simulink model "c_ep_approx_bias"  (R2024b)
settings: Solver=VariableStepAuto  StartTime=0.0  StopTime=2000  RelTol=1e-3
settings Model: Creator=merlin  LastModifiedBy=merlin

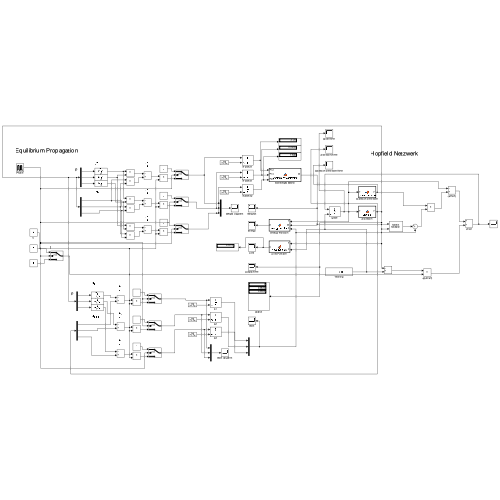
[thumbnail: Simulink's stored preview of the top-level diagram]
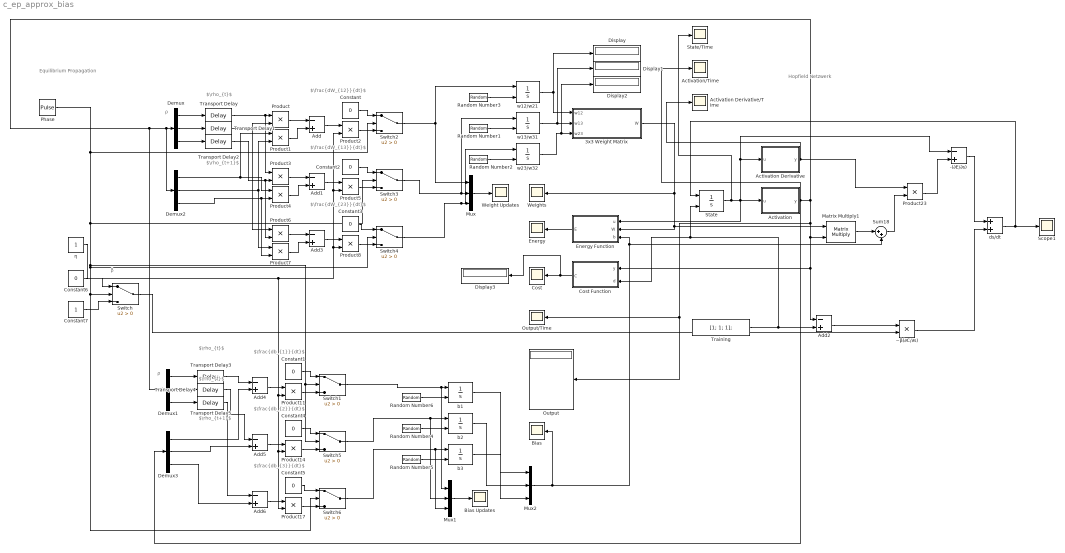
== system c_ep_approx_bias ==
  note: ρ
  note: β
  note: Equilibrium Propagation
  note: Hopfield Netzwerk
  note: $\frac{dW_{12}}{dt}$
  note: $\rho_{t}$
  note: $\rho_{t+1}$
  note: $\frac{dW_{13}}{dt}$
  note: $\frac{dW_{23}}{dt}$
  note: $\rho_{t}$
  note: $\frac{db_{2}}{dt}$
  note: ρ
  note: $\rho_{t+1}$
  note: $\frac{db_{1}}{dt}$
  note: $\frac{db_{3}}{dt}$
  note: $\rho_{t}$
  -(∂E/∂s) : Sum  Inputs=-+
  3x3 Weight Matrix : MATLAB Function  TreatAsAtomicUnit=on
  Activation : MATLAB Function  TreatAsAtomicUnit=on
  Activation Derivative : MATLAB Function  TreatAsAtomicUnit=on
  Activation Derivative/Time : Scope
  Activation/Time : Scope
  Add{,1..6} (7 alike) : Sum  Inputs=-+
  Bias : Scope
  Bias Updates : Scope
  Constant{,1..6} (7 alike) : Constant  Value=0
  Constant7 : Constant
  Cost : Scope
  Cost Function : MATLAB Function  TreatAsAtomicUnit=on
  Demux{,1..3} (4 alike) : Demux  Outputs=3
  Display{,1..3} (4 alike) : Display
  Energy : Scope
  Energy Function : MATLAB Function  TreatAsAtomicUnit=on
  Matrix Multiply1 : Product  Multiplication=Matrix(*)
  Mux : Mux  Inputs=3
  Mux1 : Mux  Inputs=3
  Mux2 : Mux  Inputs=3
  Output : Display
  Output/Time : Scope
  Phase : DiscretePulseGenerator  PulseType=Time based  Period=20  PulseWidth=50
  Product{,1..8,11,14,17,23} (13 alike) : Product
  Random Number1 : RandomNumber  Seed=13  SampleTime=0.1
  Random Number2 : RandomNumber  Seed=23  SampleTime=0.1
  Random Number3 : RandomNumber  Seed=12  SampleTime=0.1
  Random Number4 : RandomNumber  Seed=992  SampleTime=0.1
  Random Number5 : RandomNumber  Seed=993  SampleTime=0.1
  Random Number6 : RandomNumber  Seed=991  SampleTime=0.1
  Scope1 : Scope
  State : Integrator  InitialConditionSource=external
  State/Time : Scope
  Sum18 : Sum  Inputs=|++
  Switch{,1..6} (7 alike) : Switch  Criteria=u2 > Threshold  SaturateOnIntegerOverflow=off  InputSameDT=off
  Training : Constant  Value=[1; 1; 1];  VectorParams1D=off
  Transport Delay{,1..5} (6 alike) : TransportDelay
  Weight Updates : Scope
  Weights : Scope
  b1 : Integrator  InitialConditionSource=external
  b2 : Integrator  InitialConditionSource=external
  b3 : Integrator  InitialConditionSource=external
  ds/dt : Sum
  w12/w21 : Integrator  InitialConditionSource=external
  w13/w31 : Integrator  InitialConditionSource=external
  w23/w32 : Integrator  InitialConditionSource=external
  η : Constant
  −β(∂C/∂s) : Product
  wires:
  Constant6/1 -> Switch/1
  Constant7/1 -> Switch/3
  Phase/1 -> Switch6/2, Switch/2, Switch4/2, Switch5/2, Switch1/2, Switch3/2, Switch2/2
  Product23/1 -> -(∂E/∂s)/2
  Energy Function/1(E) -> Energy/1
  −β(∂C/∂s)/1 -> ds/dt/2
  Cost Function/1(C) -> Display3/1, Cost/1
  3x3 Weight Matrix/1(W) -> Weights/1, Energy Function/2(W), Matrix Multiply1/1
  w12/w21/1 -> 3x3 Weight Matrix/1(w12), Display/1
  ds/dt/1 -> Scope1/1, State/1
  Training/1 -> Cost Function/2(d), State/2, Add2/2
  -(∂E/∂s)/1 -> ds/dt/1
  Add2/1 -> −β(∂C/∂s)/1
  Sum18/1 -> Product23/2
  Matrix Multiply1/1 -> Sum18/1
  Activation Derivative/1(y) -> Activation Derivative/Time/1, Product23/1
  State/1 -> State/Time/1, Activation/1(u), Energy Function/1(u), -(∂E/∂s)/1, Activation Derivative/1(u)
  Activation/1(y) -> Demux3/1, Add2/1, Cost Function/1(y), Matrix Multiply1/2, Output/1, Output/Time/1, Demux2/1, Demux/1, Demux1/1, Activation/Time/1
  Switch/1 -> −β(∂C/∂s)/2
  w13/w31/1 -> Display1/1, 3x3 Weight Matrix/2(w13)
  w23/w32/1 -> Display2/1, 3x3 Weight Matrix/3(w23)
  Mux/1 -> Weight Updates/1
  Demux/1 -> Transport Delay/1
  Demux/2 -> Transport Delay1/1
  Demux/3 -> Transport Delay2/1
  η/1 -> Product5/2, Product2/2, Product8/2, Product17/2, Product14/2, Product11/2
  Product/1 -> Add/1
  Product1/1 -> Add/2
  Add/1 -> Product2/1
  Product2/1 -> Switch2/3
  Constant/1 -> Switch2/1
  Product3/1 -> Add1/1
  Product4/1 -> Add1/2
  Add1/1 -> Product5/1
  Product5/1 -> Switch3/3
  Constant2/1 -> Switch3/1
  Product6/1 -> Add3/1
  Product7/1 -> Add3/2
  Add3/1 -> Product8/1
  Product8/1 -> Switch4/3
  Constant3/1 -> Switch4/1
  Transport Delay/1 -> Product3/1, Product/1
  Transport Delay1/1 -> Product6/1, Product/2
  Transport Delay2/1 -> Product6/2, Product3/2
  Demux2/1 -> Product4/1, Product1/1
  Demux2/2 -> Product7/1, Product1/2
  Demux2/3 -> Product4/2, Product7/2
  Switch2/1 -> w12/w21/1, Mux/1
  Switch3/1 -> w13/w31/1, Mux/2
  Switch4/1 -> w23/w32/1, Mux/3
  Random Number3/1 -> w12/w21/2
  Random Number1/1 -> w13/w31/2
  Random Number2/1 -> w23/w32/2
  Add6/1 -> Product17/1
  Demux1/1 -> Transport Delay3/1
  Constant4/1 -> Switch5/1
  Demux1/3 -> Transport Delay5/1
  Constant1/1 -> Switch1/1
  Demux1/2 -> Transport Delay4/1
  Product11/1 -> Switch1/3
  Add4/1 -> Product11/1
  Product17/1 -> Switch6/3
  Product14/1 -> Switch5/3
  Add5/1 -> Product14/1
  Constant5/1 -> Switch6/1
  Transport Delay3/1 -> Add4/1
  Demux3/1 -> Add4/2
  Transport Delay4/1 -> Add5/1
  Demux3/2 -> Add5/2
  Transport Delay5/1 -> Add6/1
  Demux3/3 -> Add6/2
  Random Number6/1 -> b1/2
  Random Number4/1 -> b2/2
  Random Number5/1 -> b3/2
  Switch1/1 -> Mux1/1, b1/1
  Switch5/1 -> b2/1, Mux1/2
  Switch6/1 -> b3/1, Mux1/3
  Mux1/1 -> Bias Updates/1
  b1/1 -> Mux2/1
  b2/1 -> Mux2/2
  b3/1 -> Mux2/3
  Mux2/1 -> Bias/1, Sum18/2, Energy Function/3(b)

== matlab function c_ep_approx_bias/3x3 Weight Matrix ==
  data: w12 input; W output; w13 input; w23 input
function W = create3x3WeightMatrix(w12, w13, w23)
    W = [0,    w12,  w13;
         w12,  0,    w23;
         w13,  w23,  0];
end

== matlab function c_ep_approx_bias/Energy Function ==
  data: u input; E output; W input; b input
function E = energy_function(u, W, b)
    rho = @(x) 1 ./ (1 + exp(-x));

    E = (1/2) * sum(u.^2) ...
        - (1/2) * sum(sum(W .* (rho(u) * rho(u)')))
        - sum(b .* rho(u));
end

== matlab function c_ep_approx_bias/Activation Derivative ==
  data: u input; y output
function y = sigmoid_derivative(u)
% Activation Function: Logistic Function
% sigmoid = 1 ./ (1 + exp(-u));
% y = sigmoid .* (1 - sigmoid);

% Activation Function: Scaled Logistic Function
sigmoid = 1 ./ (1 + exp(-4 * u));
y = 4 .* sigmoid .* (1 - sigmoid);

% Activation Function: tanh
% y = 2 .* (1 - tanh(2 .* u).^2);

% Activation Function: ReLU
% y = double(u > 0);
end

== matlab function c_ep_approx_bias/Activation ==
  data: u input; y output
function y = sigmoid(u)
% Activation Function: Logistic Function
% y = 1 ./ (1 + exp(-u));

% Activation Function: Scaled Logistic Function
y = 1 ./ (1 + exp(-4 * u));

% Activation Function: tanh
% y = tanh(2 .* u);

% Activation Function: ReLU
y = max(u, 0);
end

== matlab function c_ep_approx_bias/Cost Function ==
  data: y input; C output; d input
function C = cost_function(y, d)
    C = 0.5 * sum((y - d).^2);
end
